simulink model "Test"  (R2022a)
settings: Solver=FixedStepAuto  StartTime=0.0  StopTime=10.0  FixedStep=0.05  RelTol=1e-3
settings Model: Creator=Stefan  LastModifiedBy=Stefan

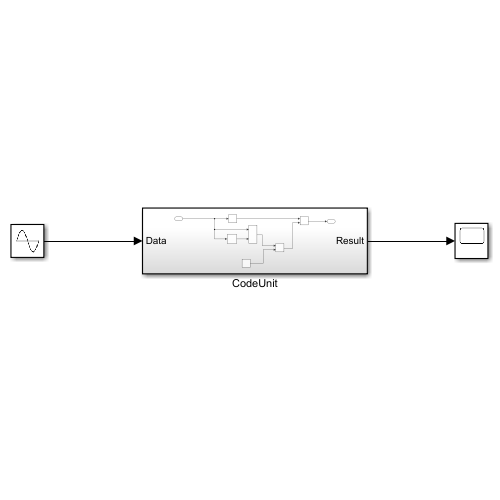
[thumbnail: Simulink's stored preview of the top-level diagram]
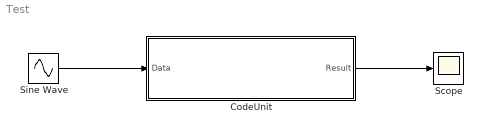
== system Test ==
  CodeUnit : Subsystem
  Scope : Scope
  Sine Wave : Sin  SampleTime=0
  wires:
  Sine Wave/1 -> CodeUnit/1(Data)
  CodeUnit/1(Result) -> Scope/1

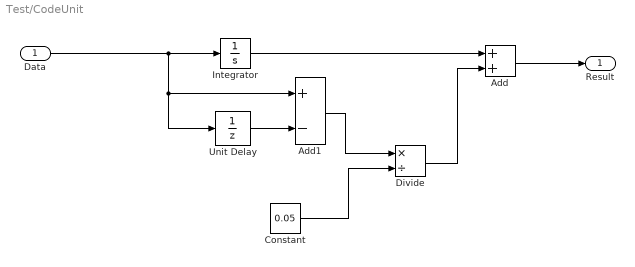
== system Test/CodeUnit ==
  Data : Inport
  Add : Sum
  Add1 : Sum  Inputs=+-
  Constant : Constant  Value=0.05
  Divide : Product  Inputs=*/
  Integrator : Integrator
  Unit Delay : UnitDelay  SampleTime=-1  HasFrameUpgradeWarning=on
  Result : Outport
  wires:
  Data/1 -> Unit Delay/1, Add1/1, Integrator/1
  Integrator/1 -> Add/1
  Divide/1 -> Add/2
  Constant/1 -> Divide/2
  Unit Delay/1 -> Add1/2
  Add1/1 -> Divide/1
  Add/1 -> Result/1
